simulink model "simulation_lab3"  (R2025b)
settings: Solver=ode45  StartTime=0.0  StopTime=10.0  MaxStep=0.001*Ts  MinStep=0.0001*Ts  RelTol=1e-3
undefined symbols (not defined in the file): DiscIntNeverNeededParam, step_value, Ts, y_delta_1, y_delta_2
libraries: cstblocks x2
settings Model: Creator=davidecovolo  LastModifiedBy=davidecovolo
settings SolverCC: InitialStep=0.0001*Ts

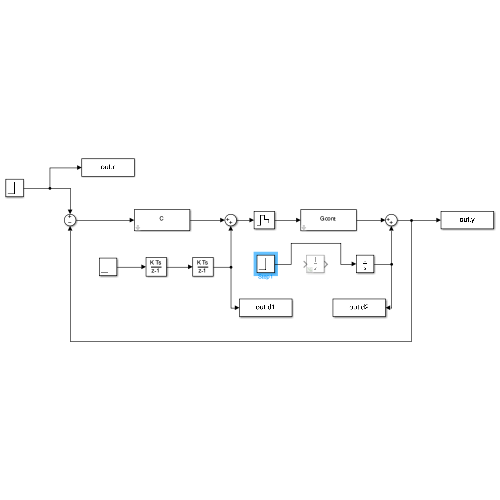
[thumbnail: Simulink's stored preview of the top-level diagram]
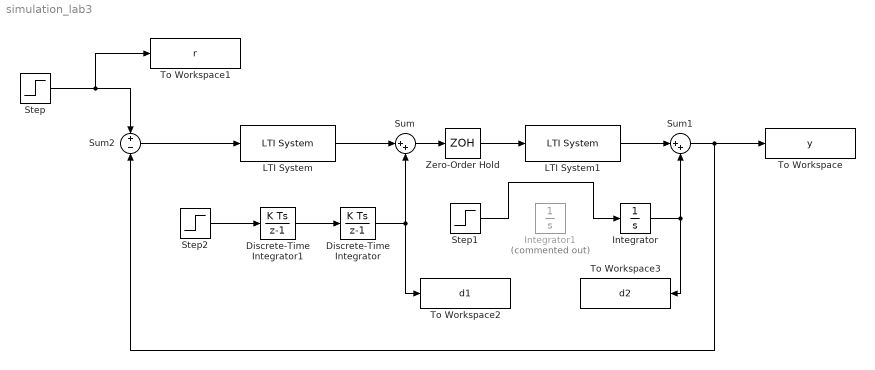
== system simulation_lab3 ==
  Discrete-Time Integrator : DiscreteIntegrator  SampleTime=Ts  ICPrevOutput=DiscIntNeverNeededParam  ICPrevScaledInput=DiscIntNeverNeededParam
  Discrete-Time Integrator1 : DiscreteIntegrator  SampleTime=Ts  ICPrevOutput=DiscIntNeverNeededParam  ICPrevScaledInput=DiscIntNeverNeededParam
  Integrator : Integrator
  Integrator1 : Integrator  Commented=on
  LTI System : cstblocks/LTI System  sys=C  IC=[]  PadeOrder=0
  LTI System1 : cstblocks/LTI System  sys=Gcont  IC=[]  PadeOrder=0
  Step : Step  Time=0  After=step_value  SampleTime=0
  Step1 : Step  Time=0  After=y_delta_2  SampleTime=0
  Step2 : Step  Time=0  After=y_delta_1  SampleTime=0
  Sum : Sum  Inputs=|++
  Sum1 : Sum  Inputs=|++
  Sum2 : Sum  Inputs=+-
  To Workspace : ToWorkspace  VariableName=y  SaveFormat=Timeseries  SampleTime=0.001*Ts
  To Workspace1 : ToWorkspace  VariableName=r  SaveFormat=Timeseries  SampleTime=0.001*Ts
  To Workspace2 : ToWorkspace  VariableName=d1  SaveFormat=Timeseries  SampleTime=Ts
  To Workspace3 : ToWorkspace  VariableName=d2  SaveFormat=Timeseries  SampleTime=0.001*Ts
  Zero-Order Hold : ZeroOrderHold  SampleTime=-1
  wires:
  Sum2/1 -> LTI System/1
  LTI System/1 -> Sum/1
  LTI System1/1 -> Sum1/1
  Sum1/1 -> To Workspace/1, Sum2/2
  Step/1 -> To Workspace1/1, Sum2/1
  Sum/1 -> Zero-Order Hold/1
  Zero-Order Hold/1 -> LTI System1/1
  Discrete-Time Integrator/1 -> Sum/2, To Workspace2/1
  Discrete-Time Integrator1/1 -> Discrete-Time Integrator/1
  Integrator/1 -> Sum1/2, To Workspace3/1
  Step2/1 -> Discrete-Time Integrator1/1
  Step1/1 -> Integrator/1
